simulink model "RK4"  (R2023b)
settings: Solver=ode4  StartTime=0.0  StopTime=100  FixedStep=0.01  RelTol=1e-3
InitFcn:
  | Ts = 0.01;
  | lon_0 = 0.959931088596881;
  | lat_0 = 0.610865238198015;
  | h_0 = 1000;
  | vn_0 = 0;
  | ve_0 = 0;
  | vd_0 = 0;
  | phi_0 = 1.2 * 0.523598775598299;
  | theta_0 = 1.2 * 0.349065850398866;
  | si_0 = 1.2 * 0.174532925199433;
  | 
  | Wbi_b = [6.939367852020717e-05;
  |          -1.852411341844020e-05;
  |          -1.139611665401531e-05];
  | Fbi_b = [3.349830943331565;
  |          -4.601792437896926;
  |          -7.970538308323724];
libraries: simulink_extras x6
settings Model: Creator=amir  LastModifiedBy=amir

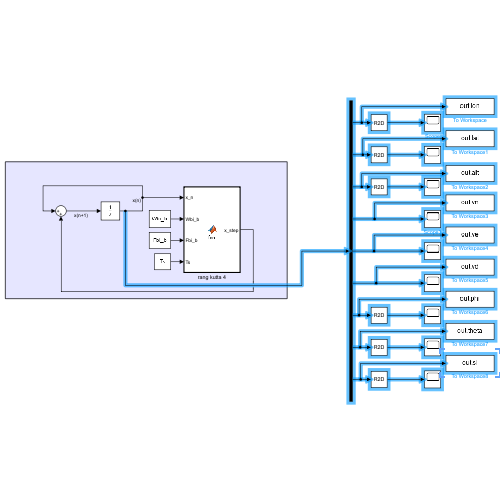
[thumbnail: Simulink's stored preview of the top-level diagram]
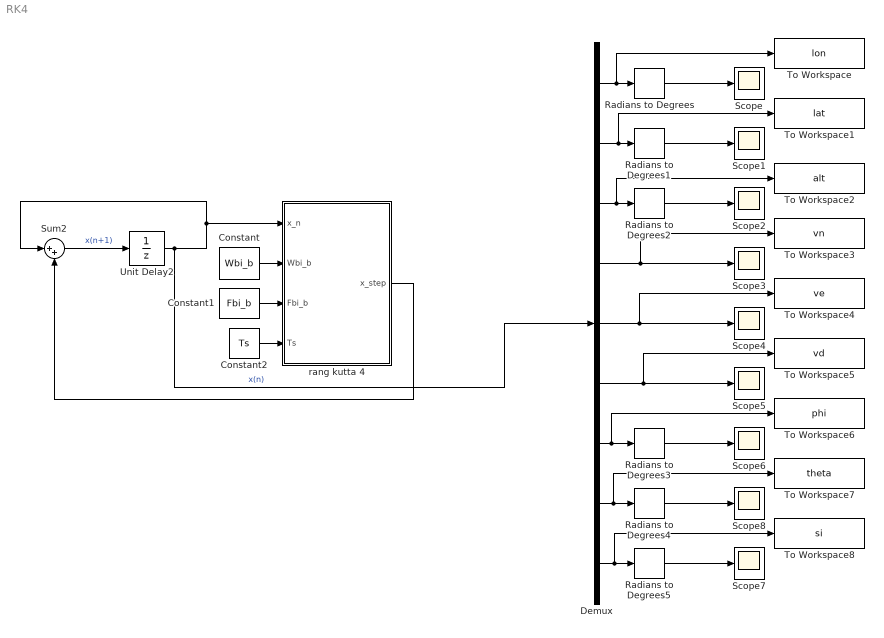
== system RK4 ==
  Constant : Constant  Value=Wbi_b
  Constant1 : Constant  Value=Fbi_b
  Constant2 : Constant  Value=Ts
  Demux : Demux  Outputs=9
  Radians to Degrees{,1..5} (6 alike) : simulink_extras/Transformations/Radians to Degrees
  Scope{,1..8} (9 alike) : Scope
  Sum2 : Sum  Inputs=|++
  To Workspace : ToWorkspace  VariableName=lon  SampleTime=-1
      settings: Save2DSignal=2-D array (concatenate along first dimension)
  To Workspace1 : ToWorkspace  VariableName=lat  SampleTime=-1
      settings: Save2DSignal=2-D array (concatenate along first dimension)
  To Workspace2 : ToWorkspace  VariableName=alt  SampleTime=-1
      settings: Save2DSignal=2-D array (concatenate along first dimension)
  To Workspace3 : ToWorkspace  VariableName=vn  SampleTime=-1
      settings: Save2DSignal=2-D array (concatenate along first dimension)
  To Workspace4 : ToWorkspace  VariableName=ve  SampleTime=-1
      settings: Save2DSignal=2-D array (concatenate along first dimension)
  To Workspace5 : ToWorkspace  VariableName=vd  SampleTime=-1
      settings: Save2DSignal=2-D array (concatenate along first dimension)
  To Workspace6 : ToWorkspace  VariableName=phi  SampleTime=-1
      settings: Save2DSignal=2-D array (concatenate along first dimension)
  To Workspace7 : ToWorkspace  VariableName=theta  SampleTime=-1
      settings: Save2DSignal=2-D array (concatenate along first dimension)
  To Workspace8 : ToWorkspace  VariableName=si  SampleTime=-1
      settings: Save2DSignal=2-D array (concatenate along first dimension)
  Unit Delay2 : UnitDelay  InitialCondition=[lon_0;lat_0;h_0;vn_0;ve_0;vd_0;phi_0;theta_0;si_0]  SampleTime=-1  HasFrameUpgradeWarning=on
  rang kutta 4 : MATLAB Function  TreatAsAtomicUnit=on
  wires:
  rang kutta 4/1(x_step) -> Sum2/2
  Constant2/1 -> rang kutta 4/4(Ts)
  Unit Delay2/1 -> Demux/1, Sum2/1, rang kutta 4/1(x_n)  "x(n)"
  Sum2/1 -> Unit Delay2/1  "x(n+1)"
  Constant/1 -> rang kutta 4/2(Wbi_b)
  Constant1/1 -> rang kutta 4/3(Fbi_b)
  Demux/1 -> To Workspace/1, Radians to Degrees/1
  Demux/2 -> To Workspace1/1, Radians to Degrees1/1
  Demux/3 -> To Workspace2/1, Radians to Degrees2/1
  Demux/4 -> To Workspace3/1, Scope3/1
  Demux/5 -> To Workspace4/1, Scope4/1
  Demux/6 -> To Workspace5/1, Scope5/1
  Demux/7 -> To Workspace6/1, Radians to Degrees3/1
  Demux/8 -> To Workspace7/1, Radians to Degrees4/1
  Demux/9 -> To Workspace8/1, Radians to Degrees5/1
  Radians to Degrees/1 -> Scope/1
  Radians to Degrees1/1 -> Scope1/1
  Radians to Degrees2/1 -> Scope2/1
  Radians to Degrees3/1 -> Scope6/1
  Radians to Degrees4/1 -> Scope8/1
  Radians to Degrees5/1 -> Scope7/1

== matlab function RK4/rang kutta 4 ==
  data: x_n input; Wbi_b input; Fbi_b input; x_step output; Ts input
function x_step = fcn(x_n, Wbi_b, Fbi_b, Ts)

dx1 = state_derivative(x_n, Wbi_b, Fbi_b) * Ts;

dx2 = state_derivative(x_n + dx1 / 2, Wbi_b, Fbi_b) * Ts;

dx3 = state_derivative(x_n + dx2 / 2, Wbi_b, Fbi_b) * Ts;

dx4 = state_derivative(x_n + dx3, Wbi_b, Fbi_b) * Ts;

x_step = (1/6) * (dx1 + 2 * dx2 + 2 * dx3 + dx4);
